simulink subsystem "Modelo"  (R2025b)
settings: Solver=VariableStepAuto  StartTime=0.0  StopTime=10.0  RelTol=1e-3
values from neighbouring files (symbols this model uses):
  b_eq = b_m + b_l/(r_m2l^2)    (= 2.19444444444e-05)    [coeficientes.m]
  g = 9.80665    [coeficientes.m]
  J_eq = J_m + J_l/(r_m2l^2)    (= 4.58263888889e-05)    [coeficientes.m]
  k_l = 0.1    [coeficientes.m]
  r_m2l = 120.0    (= 120)    [coeficientes.m]
settings Model: Creator=barrios14101  LastModifiedBy=barrios14101

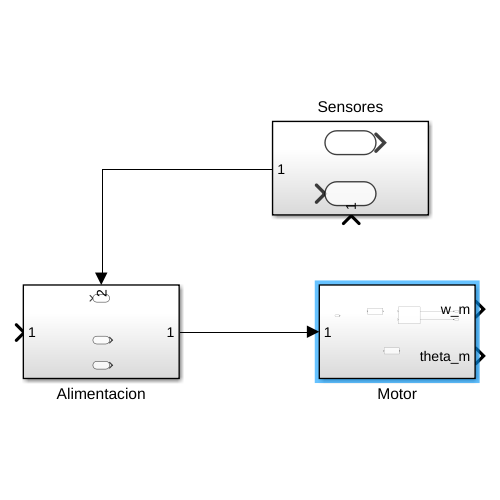
[thumbnail: Simulink's stored preview of the top-level diagram]
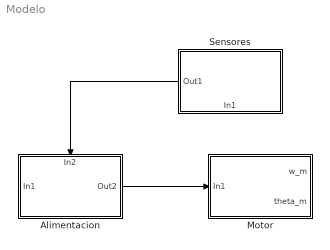
== system Modelo ==
  Alimentacion : Subsystem
      settings: PortSchema="{\"entries\":[{\"content\":{\"sides\":[{\"content\":{\"connectorIds\":[\"In1\"]},\"type\":\"ConnectorPlacement.EquallySpacedRectSide\",\"uuid\":\"0c953847-a542-44e1-afa1-eb16e3fe163f\"},{\"content\":{\"connectorIds\":[\"Out1\"],\"side\":\"RIGHT\"},\"type\":\"ConnectorPlacement.EquallySpacedRectSide\",\"uuid\":\"d6f8d29b-16c5-463f-b013-7003ed613fe0\"},{\"content\":{\"connectorIds\":[\"In2\"],\"side\":\"TOP\"},\"type\":\"ConnectorPlacement.EquallySpacedRectSide\",\"uuid\":\"60c3fb2f-c7a9-4bb3-be2b-510700c2fe0f\"},{\"content\":{\"side\":\"BOTTOM\"},\"type\":\"ConnectorPlacement.EquallySpacedRectSide\",\"uuid\":\"5571030c-c37f-4b87-b6e8-9288f1bd1f58\"}]},\"type\":\"ConnectorPlacement.EquallySpacedConnector\",\"uuid\":\"8bfbadc8-fb17-4150-9925-c98e8d49e11f\"}],\"packageUris\":[\"http://schema.mathworks.com/mf0/Connector/R2020b\"],\"version\":\"1.0\"}"
  Motor : Subsystem
  Sensores : Subsystem
      settings: PortSchema="{\"entries\":[{\"content\":{\"sides\":[{\"content\":{\"connectorIds\":[\"Out1\"]},\"type\":\"ConnectorPlacement.EquallySpacedRectSide\",\"uuid\":\"0c953847-a542-44e1-afa1-eb16e3fe163f\"},{\"content\":{\"side\":\"RIGHT\"},\"type\":\"ConnectorPlacement.EquallySpacedRectSide\",\"uuid\":\"d6f8d29b-16c5-463f-b013-7003ed613fe0\"},{\"content\":{\"side\":\"TOP\"},\"type\":\"ConnectorPlacement.EquallySpacedRectSide\",\"uuid\":\"60c3fb2f-c7a9-4bb3-be2b-510700c2fe0f\"},{\"content\":{\"connectorIds\":[\"In1\"],\"side\":\"BOTTOM\"},\"type\":\"ConnectorPlacement.EquallySpacedRectSide\",\"uuid\":\"48731a4e-21f3-48a9-965b-1bc0b841acdd\"}]},\"type\":\"ConnectorPlacement.EquallySpacedConnector\",\"uuid\":\"8bfbadc8-fb17-4150-9925-c98e8d49e11f\"}],\"packageUris\":[\"http://schema.mathworks.com/mf0/Connector/R2020b\"],\"version\":\"1.0\"}"
  wires:
  Alimentacion/1(Out2) -> Motor/1(In1)
  Sensores/1(Out1) -> Alimentacion/2(In2)

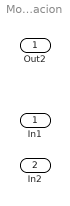
== system Modelo/Alimentacion ==
  In1 : Inport
  In2 : Inport  Port=2
  Out2 : Outport

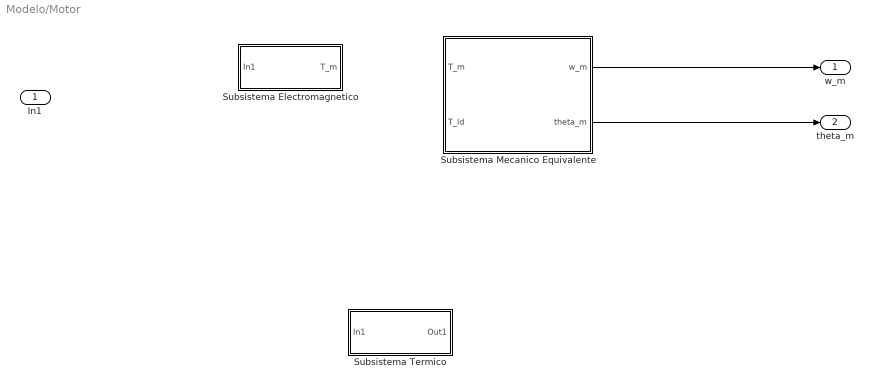
== system Modelo/Motor ==
  In1 : Inport
  Subsistema Electromagnetico : Subsystem
  Subsistema Mecanico Equivalente : Subsystem
  Subsistema Termico : Subsystem
  w_m : Outport
  theta_m : Outport  Port=2
  wires:
  Subsistema Mecanico Equivalente/1(w_m) -> w_m/1
  Subsistema Mecanico Equivalente/2(theta_m) -> theta_m/1

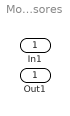
== system Modelo/Sensores ==
  In1 : Inport
  Out1 : Outport

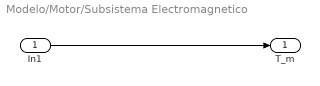
== system Modelo/Motor/Subsistema Electromagnetico ==
  In1 : Inport
  T_m : Outport
  wires:
  In1/1 -> T_m/1

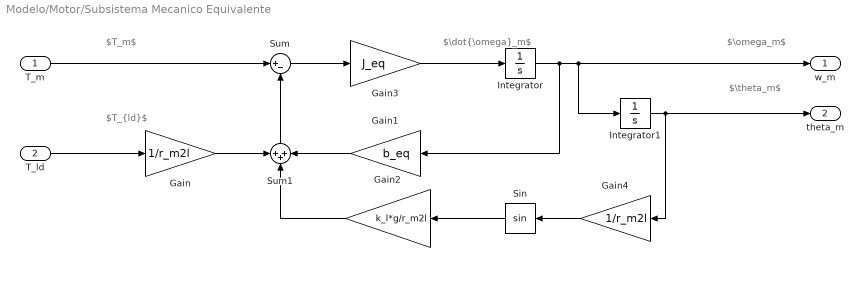
== system Modelo/Motor/Subsistema Mecanico Equivalente ==
  note: $T_m$
  note: $T_{ld}$
  note: $\dot{\omega}_m$
  note: $\omega_m$
  note: $\theta_m$
  T_m : Inport
  T_ld : Inport  Port=2
  Gain : Gain  Gain=1/r_m2l
  Gain1 : Gain  Gain=b_eq
  Gain2 : Gain  Gain=k_l*g/r_m2l
  Gain3 : Gain  Gain=J_eq
  Gain4 : Gain  Gain=1/r_m2l
  Integrator : Integrator
  Integrator1 : Integrator
  Sin : Trigonometry
  Sum : Sum  Inputs=|+-
  Sum1 : Sum  Inputs=+++
  w_m : Outport
  theta_m : Outport  Port=2
  wires:
  Integrator/1 -> Integrator1/1, w_m/1, Gain1/1
  Integrator1/1 -> theta_m/1, Gain4/1
  Sum/1 -> Gain3/1
  T_m/1 -> Sum/1
  Sum1/1 -> Sum/2
  Gain2/1 -> Sum1/2
  Gain/1 -> Sum1/1
  Sin/1 -> Gain2/1
  Gain1/1 -> Sum1/3
  Gain3/1 -> Integrator/1
  Gain4/1 -> Sin/1
  T_ld/1 -> Gain/1

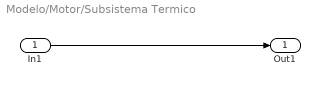
== system Modelo/Motor/Subsistema Termico ==
  In1 : Inport
  Out1 : Outport
  wires:
  In1/1 -> Out1/1
